simulink model "dc_motorParamSweep"  (R2015b)
settings: Solver=ode45  SolverMode=SingleTasking  StartTime=0.0  StopTime=10.0  RelTol=1e-3
PreLoadFcn:
  | Load_parameters
values from neighbouring files (symbols this model uses):
  R = 4.3    [Load_parameters.m]    (also in SolutionExerciseMotorParamSweep.m = Rgrid(k); motorParamSweep.m = R_values(k))
libraries: simulink x1
settings Model: RequirementInfo={'other' 'motor_reqs.doc' '@inp_scl_1' 'true' 'The model shall represent the dynamics of equations:' '' ; 'other' 'motor_reqs.doc' '@inp_scl_2' 'true' 'The model shall be parameterized. for J, L, R, b, & K,' '' ; 'other' 'motor_reqs.doc' '@inp_scl_1' 'true' 'The model shall represent the dynamics of equations: i = (1/L)((V – K(? – i(R) dt' '' } %GIDa_c543596b_ec0a_4932_b3ae_f63b6de72bba  Creator=gpacitti  LastModifiedBy=knunna
settings DataIOCC: SaveFormat=Array
settings OptimizationCC: BlockReduction=off  BooleanDataType=off
settings DebuggingCC: SaveWithParameterizedLinksMsg=none  SignalResolutionControl=TryResolveAllWithWarning
settings HardwareCC: ProdBitPerPointer=32  ProdLargestAtomicFloat=None  ProdIntDivRoundTo=Undefined  ProdEndianess=Unspecified  ProdWordSize=32  ProdHWDeviceType=32-bit Generic  TargetUnknown=on
settings GRTTargetCC: GeneratePreprocessorConditionals=Disable all
settings ConfigComp: CovModelRefEnable=Off  CovSFcnEnable=off

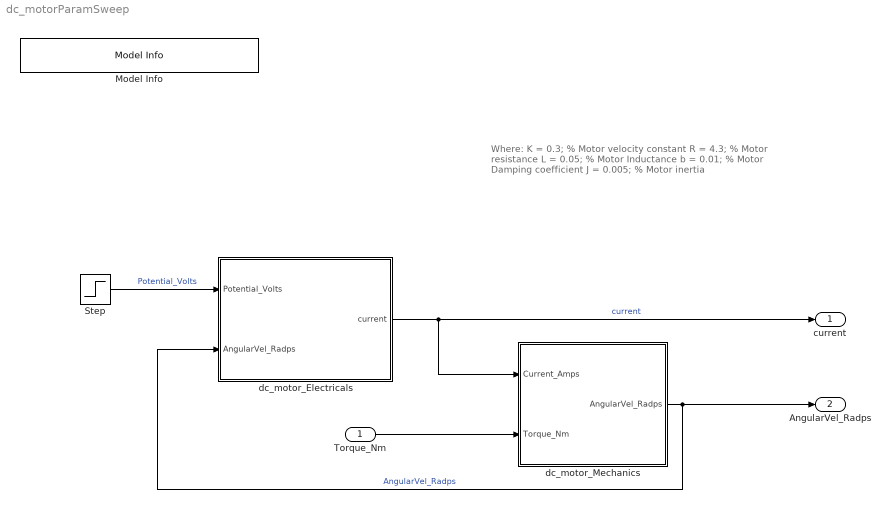
== system dc_motorParamSweep ==
  note: Where:
      | K = 0.3;	% Motor velocity constant
      | R = 4.3;	% Motor resistance
      | L = 0.05;	% Motor Inductance
      | b = 0.01;	% Motor Damping coefficient
      | J = 0.005;	% Motor inertia
  Torque_Nm : Inport
  Model Info : simulink/Model-Wide Utilities/Model Info  Frame=on  DisplayStringWithTags=Copyright 2014 The MathWorks, Inc.  HorizontalTextAlignment=Center  LeftAlignmentValue=0.5  SourceBlockDiagram=dc_motorParamSweep  TagMaxNumber=20
  Step : Step  Before=0.2  After=5  SampleTime=0
  dc_motor_Electricals : Subsystem
  dc_motor_Mechanics : Subsystem
  "current " : Outport
  AngularVel_Radps : Outport  Port=2
  wires:
  Step/1 -> dc_motor_Electricals/1(Potential_Volts)  "Potential_Volts"
  dc_motor_Mechanics/1(AngularVel_Radps) -> dc_motor_Electricals/2(AngularVel_Radps), AngularVel_Radps/1  "AngularVel_Radps"
  dc_motor_Electricals/1("current ") -> "current "/1, dc_motor_Mechanics/1(Current_Amps)  "current"
  Torque_Nm/1 -> dc_motor_Mechanics/2(Torque_Nm)

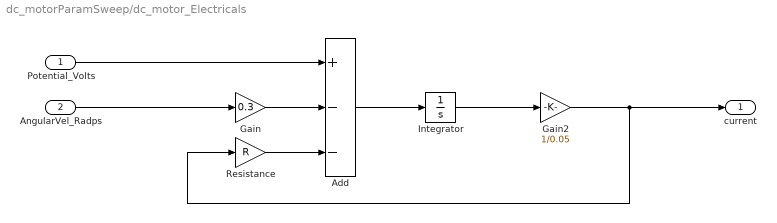
== system dc_motorParamSweep/dc_motor_Electricals ==
  Potential_Volts : Inport
  AngularVel_Radps : Inport  Port=2
  Add : Sum  Inputs=+--
  Gain : Gain  Gain=0.3
  Gain2 : Gain  Gain=1/0.05
  Integrator : Integrator
  Resistance : Gain  Gain=R
  "current " : Outport
  wires:
  Gain2/1 -> "current "/1, Resistance/1
  Integrator/1 -> Gain2/1
  Resistance/1 -> Add/3
  Potential_Volts/1 -> Add/1
  Gain/1 -> Add/2
  Add/1 -> Integrator/1
  AngularVel_Radps/1 -> Gain/1

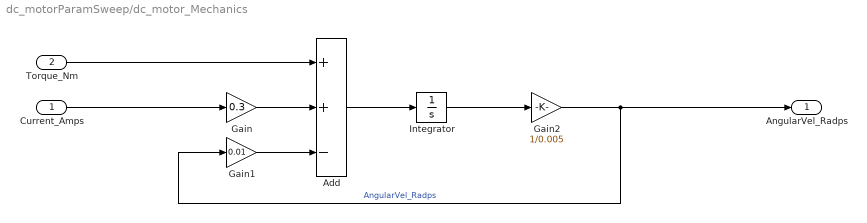
== system dc_motorParamSweep/dc_motor_Mechanics ==
  Current_Amps : Inport
  Torque_Nm : Inport  Port=2
  Add : Sum  Inputs=++-
  Gain : Gain  Gain=0.3
  Gain1 : Gain  Gain=0.01
  Gain2 : Gain  Gain=1/0.005
  Integrator : Integrator
  AngularVel_Radps : Outport
  wires:
  Gain2/1 -> AngularVel_Radps/1, Gain1/1  "AngularVel_Radps"
  Integrator/1 -> Gain2/1
  Gain1/1 -> Add/3
  Torque_Nm/1 -> Add/1
  Gain/1 -> Add/2
  Add/1 -> Integrator/1
  Current_Amps/1 -> Gain/1
